simulink model "lab4_1"  (R2023b)
settings: Solver=FixedStepAuto  StartTime=0.0  StopTime=10.0  FixedStep=0.001  RelTol=1e-3
undefined symbols (not defined in the file): a_0, a_1, a_2
settings Model: Creator=nsukh  LastModifiedBy=nsukh

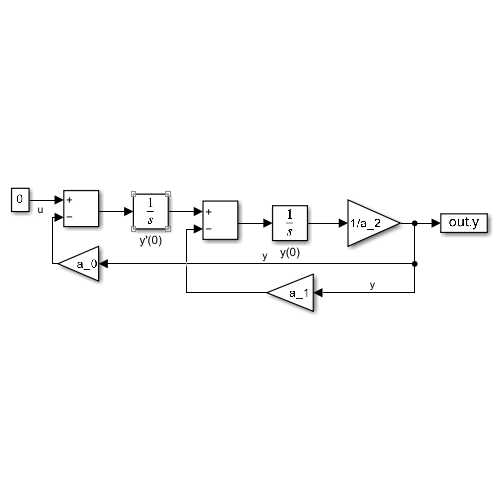
[thumbnail: Simulink's stored preview of the top-level diagram]
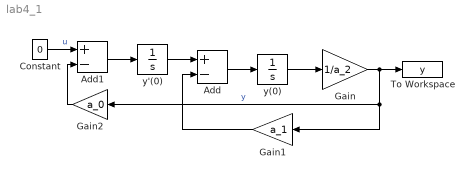
== system lab4_1 ==
  Add : Sum  Inputs=+-
  Add1 : Sum  Inputs=+-
  Constant : Constant  Value=0
  Gain : Gain  Gain=1/a_2
  Gain1 : Gain  Gain=a_1
  Gain2 : Gain  Gain=a_0
  To Workspace : ToWorkspace  VariableName=y  SaveFormat=Timeseries  SampleTime=-1
  y'(0) : Integrator  InitialCondition=4
  y(0) : Integrator
  wires:
  y(0)/1 -> Gain/1
  Gain/1 -> To Workspace/1, Gain1/1, Gain2/1  "y"
  Add/1 -> y(0)/1
  Gain1/1 -> Add/2
  y'(0)/1 -> Add/1
  Add1/1 -> y'(0)/1
  Gain2/1 -> Add1/2
  Constant/1 -> Add1/1  "u"
